simulink model "UniControlSystem"  (R2015a)
settings: Solver=ode1  SolverMode=SingleTasking  StartTime=0.0  StopTime=10.0  FixedStep=0.01  RelTol=1e-3
values from neighbouring files (symbols this model uses):
  Phi_PID_D = 0    [UniControlSystem.mat]
  Phi_PID_I = 0    [UniControlSystem.mat]
  Phi_PID_P = 0    [UniControlSystem.mat]
  Position = 0    [UniControlSystem.mat]
  x_PID_D = 0    [UniControlSystem.mat]
  x_PID_HLIM = 9    [UniControlSystem.mat]
  x_PID_I = 0    [UniControlSystem.mat]
  x_PID_LLIM = -9    [UniControlSystem.mat]
  x_PID_P = 0    [UniControlSystem.mat]
libraries: simulink x2
settings Model: TunableVars=Phi_PID_D,Phi_PID_I,Phi_PID_P,Position,x_PID_D,x_PID_HLIM,x_PID_I,x_PID_LLIM,x_PID_P  TunableVarsStorageClass=ExportedGlobal,ExportedGlobal,ExportedGlobal,ExportedGlobal,ExportedGlobal,ExportedGlobal,ExportedGlobal,ExportedGlobal,ExportedGlobal  TunableVarsTypeQualifier=,,,,,,,,  Creator=Roman Grewenig  LastModifiedBy=grewenig
settings DataIOCC: LimitDataPoints=off  SaveOutput=off  SignalLogging=off  DSMLogging=off  VisualizeSimOutput=off  SaveTime=off
settings OptimizationCC: BlockReduction=off  StateBitsets=on  DataBitsets=on  NoFixptDivByZeroProtection=on  EfficientFloat2IntCast=on  OptimizeModelRefInitCode=on  LifeSpan=1  MaxStackSize=64
settings DebuggingCC: UnconnectedOutputMsg=none  UnknownTsInhSupMsg=error
settings HardwareCC: ProdLargestAtomicInteger=Long  ProdLargestAtomicFloat=Double  ProdEndianess=LittleEndian  ProdHWDeviceType=ARM Compatible->ARM Cortex
settings RTWCC: SystemTargetFile=ert.tlc  GenCodeOnly=on  TemplateMakefile=ert_default_tmf  Description=Embedded Coder  GenerateReport=on  RTWVerbose=off  IncludeHyperlinkInReport=on  LaunchReport=on  GenerateTraceInfo=on  GenerateTraceReport=on  GenerateTraceReportSl=on  GenerateTraceReportSf=on  GenerateTraceReportEml=on
settings CodeAppCC: ForceParamTrailComments=on  IgnoreCustomStorageClasses=off  SimulinkDataObjDesc=on  CustomSymbolStrGlobalVar=rt$N$M  CustomSymbolStrType=$N$M  CustomSymbolStrFcn=$N$M$F  CustomSymbolStrMacro=$N$M  ParamNamingRule=UpperCase  InsertBlockDesc=on
settings ERTTargetCC: GenerateSampleERTMain=off  ParMdlRefBuildCompliant=on  CompOptLevelCompliant=on  ConcurrentExecutionCompliant=on  IncludeMdlTerminateFcn=off  ERTFirstTimeCompliant=on  SupportNonFinite=off  SupportComplex=off  SupportContinuousTime=off  SupportVariableSizeSignals=off  ModelStepFunctionPrototypeControlCompliant=on  CPPClassGenCompliant=on  InlinedParameterPlacement=Hierarchical  ERTCustomFileTemplate=example_file_process.tlc  ERTFilePackagingFormat=Compact
settings ConfigComp: Description=Polyspace Custom Configuration Component  PSAutoStubLUT=off

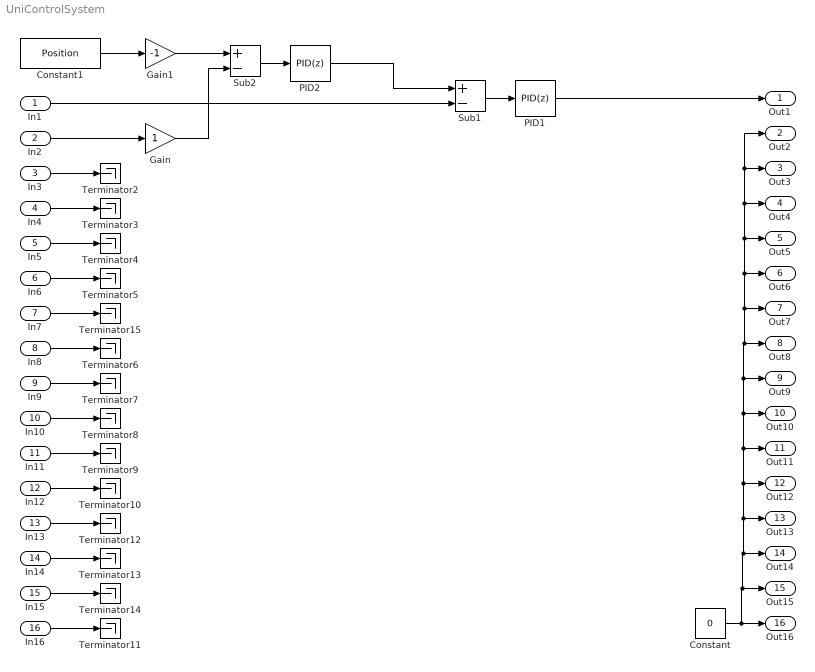
== system UniControlSystem ==
  In1 : Inport  OutDataTypeStr=double
  In2 : Inport  Port=2  OutDataTypeStr=double
  In3 : Inport  Port=3  OutDataTypeStr=double
  In4 : Inport  Port=4  OutDataTypeStr=double
  In5 : Inport  Port=5  OutDataTypeStr=double
  In6 : Inport  Port=6  OutDataTypeStr=double
  In7 : Inport  Port=7  OutDataTypeStr=double
  In8 : Inport  Port=8  OutDataTypeStr=double
  In9 : Inport  Port=9  OutDataTypeStr=double
  In10 : Inport  Port=10  OutDataTypeStr=double
  In11 : Inport  Port=11  OutDataTypeStr=double
  In12 : Inport  Port=12  OutDataTypeStr=double
  In13 : Inport  Port=13  OutDataTypeStr=double
  In14 : Inport  Port=14  OutDataTypeStr=double
  In15 : Inport  Port=15  OutDataTypeStr=double
  In16 : Inport  Port=16  OutDataTypeStr=double
  Constant : Constant  Value=0
  Constant1 : Constant  Value=Position
  Gain : Gain
  Gain1 : Gain  Gain=-1
  PID1 : simulink/Continuous/PID Controller  Controller=PID  TimeDomain=Discrete-time  SampleTime=0.01  IntegratorMethod=Forward Euler  FilterMethod=Forward Euler  Form=Parallel  UseFilter=on  ControllerParametersSource=internal  P=Phi_PID_P  I=Phi_PID_I  D=Phi_PID_D  N=10  InitialConditionSource=internal  InitialConditionForIntegrator=0  InitialConditionForFilter=0  ExternalReset=none  LimitOutput=on  UpperSaturationLimit=2  LowerSaturationLimit=-2  LinearizeAsGain=off  AntiWindupMode=clamping  Kb=1  TrackingMode=off  Kt=1  PParamMin=[]  PParamMax=[]  IParamMin=[]  IParamMax=[]  DParamMin=[]  DParamMax=[]  NParamMin=[]  NParamMax=[]  KbParamMin=[]  KbParamMax=[]  KtParamMin=[]  KtParamMax=[]  POutMin=[]  POutMax=[]  IOutMin=[]  IOutMax=[]  DOutMin=[]  DOutMax=[]  NOutMin=[]  NOutMax=[]  KbOutMin=[]  KbOutMax=[]  KtOutMin=[]  KtOutMax=[]  IntegratorOutMin=[]  IntegratorOutMax=[]  FilterOutMin=[]  FilterOutMax=[]  SumOutMin=[]  SumOutMax=[]  SumI1OutMin=[]  SumI1OutMax=[]  SumI2OutMin=[]  SumI2OutMax=[]  SumI3OutMin=[]  SumI3OutMax=[]  SumDOutMin=[]  SumDOutMax=[]  SaturationOutMin=[]  SaturationOutMax=[]  IntegratorContinuousStateAttributes=''  IntegratorStateMustResolveToSignalObject=off  IntegratorRTWStateStorageClass=Auto  FilterContinuousStateAttributes=''  FilterStateMustResolveToSignalObject=off  FilterRTWStateStorageClass=Auto  DifferentiatorICPrevScaledInput=0  DifferentiatorOutMin=[]  DifferentiatorOutMax=[]
  PID2 : simulink/Continuous/PID Controller  Controller=PID  TimeDomain=Discrete-time  SampleTime=0.01  IntegratorMethod=Forward Euler  FilterMethod=Forward Euler  Form=Parallel  UseFilter=on  ControllerParametersSource=internal  P=x_PID_P  I=x_PID_I  D=x_PID_D  N=1  InitialConditionSource=internal  InitialConditionForIntegrator=0  InitialConditionForFilter=0  ExternalReset=none  LimitOutput=on  UpperSaturationLimit=x_PID_HLIM  LowerSaturationLimit=x_PID_LLIM  LinearizeAsGain=off  AntiWindupMode=clamping  Kb=1  TrackingMode=off  Kt=1  PParamMin=[]  PParamMax=[]  IParamMin=[]  IParamMax=[]  DParamMin=[]  DParamMax=[]  NParamMin=[]  NParamMax=[]  KbParamMin=[]  KbParamMax=[]  KtParamMin=[]  KtParamMax=[]  POutMin=[]  POutMax=[]  IOutMin=[]  IOutMax=[]  DOutMin=[]  DOutMax=[]  NOutMin=[]  NOutMax=[]  KbOutMin=[]  KbOutMax=[]  KtOutMin=[]  KtOutMax=[]  IntegratorOutMin=[]  IntegratorOutMax=[]  FilterOutMin=[]  FilterOutMax=[]  SumOutMin=[]  SumOutMax=[]  SumI1OutMin=[]  SumI1OutMax=[]  SumI2OutMin=[]  SumI2OutMax=[]  SumI3OutMin=[]  SumI3OutMax=[]  SumDOutMin=[]  SumDOutMax=[]  SaturationOutMin=[]  SaturationOutMax=[]  IntegratorContinuousStateAttributes=''  IntegratorStateMustResolveToSignalObject=off  IntegratorRTWStateStorageClass=Auto  FilterContinuousStateAttributes=''  FilterStateMustResolveToSignalObject=off  FilterRTWStateStorageClass=Auto  DifferentiatorICPrevScaledInput=0  DifferentiatorOutMin=[]  DifferentiatorOutMax=[]
  Sub1 : Sum  Inputs=+-
  Sub2 : Sum  Inputs=+-
  Terminator{2..15} (14 alike) : Terminator
  Out1 : Outport  OutDataTypeStr=double
  Out2 : Outport  Port=2  OutDataTypeStr=double  SampleTime=0.01
  Out3 : Outport  Port=3  OutDataTypeStr=double  SampleTime=0.01
  Out4 : Outport  Port=4  OutDataTypeStr=double  SampleTime=0.01
  Out5 : Outport  Port=5  OutDataTypeStr=double  SampleTime=0.01
  Out6 : Outport  Port=6  OutDataTypeStr=double  SampleTime=0.01
  Out7 : Outport  Port=7  OutDataTypeStr=double  SampleTime=0.01
  Out8 : Outport  Port=8  OutDataTypeStr=double  SampleTime=0.01
  Out9 : Outport  Port=9  OutDataTypeStr=double  SampleTime=0.01
  Out10 : Outport  Port=10  OutDataTypeStr=double  SampleTime=0.01
  Out11 : Outport  Port=11  OutDataTypeStr=double  SampleTime=0.01
  Out12 : Outport  Port=12  OutDataTypeStr=double  SampleTime=0.01
  Out13 : Outport  Port=13  OutDataTypeStr=double  SampleTime=0.01
  Out14 : Outport  Port=14  OutDataTypeStr=double  SampleTime=0.01
  Out15 : Outport  Port=15  OutDataTypeStr=double  SampleTime=0.01
  Out16 : Outport  Port=16  OutDataTypeStr=double  SampleTime=0.01
  wires:
  In8/1 -> Terminator6/1
  In9/1 -> Terminator7/1
  In10/1 -> Terminator8/1
  In11/1 -> Terminator9/1
  In12/1 -> Terminator10/1
  In13/1 -> Terminator12/1
  In14/1 -> Terminator13/1
  In15/1 -> Terminator14/1
  In16/1 -> Terminator11/1
  Sub1/1 -> PID1/1
  In6/1 -> Terminator5/1
  In5/1 -> Terminator4/1
  In4/1 -> Terminator3/1
  In3/1 -> Terminator2/1
  In7/1 -> Terminator15/1
  In1/1 -> Sub1/2
  Sub2/1 -> PID2/1
  PID2/1 -> Sub1/1
  Constant/1 -> Out6/1, Out5/1, Out4/1, Out3/1, Out2/1, Out7/1, Out8/1, Out9/1, Out10/1, Out11/1, Out12/1, Out13/1, Out14/1, Out15/1, Out16/1
  In2/1 -> Gain/1
  Gain/1 -> Sub2/2
  Constant1/1 -> Gain1/1
  Gain1/1 -> Sub2/1
  PID1/1 -> Out1/1
